simulink model "Cart_Pendulum_n9945008"  (R2018b)
settings: Solver=VariableStepAuto  StartTime=0.0  StopTime=10.0  RelTol=1e-3
values from neighbouring files (symbols this model uses):
  g = 9.81    [MainFile_Linearised_a_n9945008.m]
  l = 0.2    [MainFile_Linearised_a_n9945008.m]
  m = 0.15    [MainFile_Linearised_a_n9945008.m]
  Mc = 0.4    [MainFile_Linearised_a_n9945008.m]
settings Model: Creator=Cody  LastModifiedBy=Cody

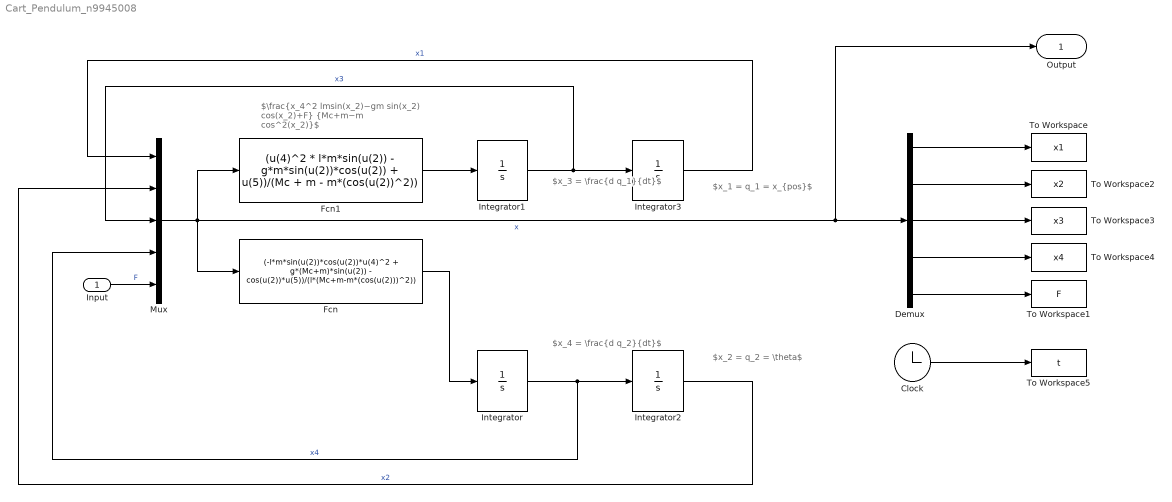
== system Cart_Pendulum_n9945008 ==
  note: $\frac{x_4^2 lmsin(x_2)−gm sin(x_2) cos(x_2)+F} {Mc+m−m cos^2(x_2)}$
  note: $x_2 = q_2 = \theta$
  note: $x_4 = \frac{d q_2}{dt}$
  note: $x_3 = \frac{d q_1}{dt}$
  note: $x_1 = q_1 = x_{pos}$
  Input : Inport
  Clock : Clock
  Demux : Demux  Outputs=5
  Fcn : Fcn  Expr=(-l*m*sin(u(2))*cos(u(2))*u(4)^2 + g*(Mc+m)*sin(u(2)) - cos(u(2))*u(5))/(l*(Mc+m-m*(cos(u(2)))^2))
  Fcn1 : Fcn  Expr=(u(4)^2 * l*m*sin(u(2)) - g*m*sin(u(2))*cos(u(2)) + u(5))/(Mc + m - m*(cos(u(2))^2))
  Integrator : Integrator
  Integrator1 : Integrator
  Integrator2 : Integrator  InitialCondition=pi/180
  Integrator3 : Integrator
  Mux : Mux  Inputs=5
  To Workspace : ToWorkspace  VariableName=x1  SampleTime=-1
      settings: Save2DSignal=2-D array (concatenate along first dimension)
  To Workspace1 : ToWorkspace  VariableName=F  SampleTime=-1
      settings: Save2DSignal=2-D array (concatenate along first dimension)
  To Workspace2 : ToWorkspace  VariableName=x2  SampleTime=-1
      settings: Save2DSignal=2-D array (concatenate along first dimension)
  To Workspace3 : ToWorkspace  VariableName=x3  SampleTime=-1
      settings: Save2DSignal=2-D array (concatenate along first dimension)
  To Workspace4 : ToWorkspace  VariableName=x4  SampleTime=-1
      settings: Save2DSignal=2-D array (concatenate along first dimension)
  To Workspace5 : ToWorkspace  VariableName=t  SampleTime=-1
      settings: Save2DSignal=2-D array (concatenate along first dimension)
  Output : Outport
  wires:
  Mux/1 -> Fcn/1, Output/1, Demux/1, Fcn1/1  "x"
  Fcn/1 -> Integrator/1
  Integrator/1 -> Mux/4, Integrator2/1  "x4"
  Integrator2/1 -> Mux/2  "x2"
  Fcn1/1 -> Integrator1/1
  Integrator1/1 -> Integrator3/1, Mux/3  "x3"
  Integrator3/1 -> Mux/1  "x1"
  Input/1 -> Mux/5  "F"
  Demux/1 -> To Workspace/1
  Demux/3 -> To Workspace3/1
  Demux/4 -> To Workspace4/1
  Demux/5 -> To Workspace1/1
  Demux/2 -> To Workspace2/1
  Clock/1 -> To Workspace5/1
